simulink model "example_Resident_Task44"  (R2018b)
settings: Solver=ode45  StartTime=0.0  StopTime=3*24*3600  MaxStep=600  RelTol=1e-4  AbsTol=1e-6  EnableMultiTasking=on
libraries: simulink x2, carnot x2
settings Model: Creator=drhf  LastModifiedBy=drhf
settings SolverCC: AutoScaleAbsTol=off  ZeroCrossAlgorithm=Adaptive
settings DataIOCC: LimitDataPoints=on  SaveFormat=Array
settings OptimizationCC: ExpressionDepthLimit=2147483647  LifeSpan=inf
settings DebuggingCC: UnderspecifiedInitializationDetection=Classic  MergeDetectMultiDrivingBlocksExec=none  SolverPrmCheckMsg=warning  StateNameClashWarn=warning  SFUnexpectedBacktrackingDiag=warning  SFNoUnconditionalDefaultTransitionDiag=warning  SFExecutionAtInitializationDiag=none
settings HardwareCC: ProdBitPerPointer=32  ProdBitPerSizeT=32  ProdBitPerPtrDiffT=32  ProdLargestAtomicFloat=None  ProdIntDivRoundTo=Undefined  ProdEndianess=Unspecified  ProdWordSize=32  ProdHWDeviceType=32-bit Generic
settings ModelReferenceCC: PropagateSignalLabelsOutOfModel=off
settings SFSimCC: SimUseLocalCustomCode=off
settings RTWCC: RTWUseLocalCustomCode=off
settings CodeAppCC: StateflowObjectComments=on
settings GRTTargetCC: TargetLangStandard=C89/C90 (ANSI)  GeneratePreprocessorConditionals=Disable all  CombineOutputUpdateFcns=off  GRTInterface=on
settings ConfigComp: CovMetricSettings=dw  CovHtmlReporting=on  CovSaveCumulativeToWorkspaceVar=on  CovSaveSingleToWorkspaceVar=on  CovExternalEMLEnable=off

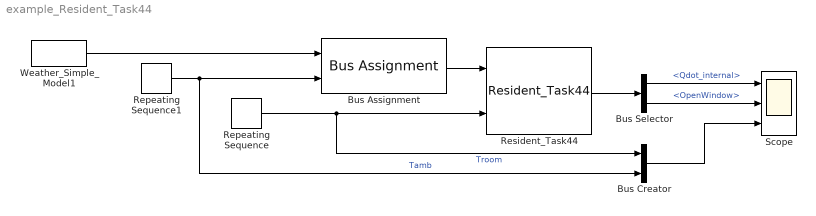
== system example_Resident_Task44 ==
  Bus Assignment : BusAssignment  AssignedSignals=Temperature_Ambient
  Bus Creator : BusCreator  Inputs=2
  Bus Selector : BusSelector  OutputSignals=Qdot_internal,OpenWindow
  Repeating Sequence : simulink/Sources/Repeating Sequence  rep_seq_t="[0  24 24.1 34 34.1 38 38.1 48 48.1 72]*3600"  rep_seq_y="[25 25 20   20  25  25  20   20  25   25]"
  Repeating Sequence1 : simulink/Sources/Repeating Sequence  rep_seq_t="[0  58 58.1 62 62.1 72]*3600"  rep_seq_y="[20 20  0    0  20    20]"
  Resident_Task44 : carnot/Load/Houses/Resident_Task44  period=24*3600  rep_seq_te=[0 1 6 7 8 9 11 12 13 18 19 20 22 23]*3600  rep_seq_de=[1 5 1 1 1 2 1 1 4 2 1 2 1 1]*3600  rep_seq_ye=[105 55 392.5 457.5 420 55 250 55 120 170 615 420 442.5 355]  rep_seq_to=[0 6 7 8 9 11 12 13 14 15 17 18 20 21 22]*3600  rep_seq_do=[6 1 1 1 2 1 1 1 1 2 1 2 1 1 2]*3600  rep_seq_yo=[4 2 3 2 0 1 3 2 1 0 1 2 4 3 4]*60  Topen=24  Tclose=23  TrAboveTa=2  TaTooCold=12  timeFIR=24  TaIni=12  starttime=8  stoptime=22  TroomShadeOn=23.8  TroomShadeOff=22.8  SolarShadeOn=300  SolarShadeOff=200  max_shade=1  CalcAirComp=on  mdotCO2=0.01  mdotH2O=0.02  mdotVOC=0.03
      settings: SourceProductName=Carnot
  Scope : Scope  NumInputPorts=3
  Weather_Simple_Model1 : carnot/Weather/Weather_Simple_Model  Ibn=900  Idg=100  tamb=5  deltaTsky=-6  rh=50  precip="10e-3/24/3600           % 10 mm in 24 h"  cloud=0.125  p=1013e2  vw=1  wdir=270  lat=-20  colangle=0  colazi=0  colrot=0
      settings: SourceProductName=Carnot
  wires:
  Repeating Sequence1/1 -> Bus Creator/2, Bus Assignment/2  "Tamb"
  Repeating Sequence/1 -> Bus Creator/1, Resident_Task44/2  "Troom"
  Weather_Simple_Model1/1 -> Bus Assignment/1
  Bus Assignment/1 -> Resident_Task44/1
  Resident_Task44/1 -> Bus Selector/1
  Bus Selector/1 -> Scope/1  "<Qdot_internal>"
  Bus Selector/2 -> Scope/2  "<OpenWindow>"
  Bus Creator/1 -> Scope/3
